simulink model "BestRun_VehicleModel_pntwo"  (R2021b)
settings: Solver=ode4  StartTime=0.0  StopTime=800  FixedStep=0.01  RelTol=1e-3  EnableMultiTasking=on
values from neighbouring files (symbols this model uses):
  Aera = 2.22    [Para_bestRun.m]
  BETT = 0.5*(0.878+0.844)*Mass*RofW    (= 426.1215567)    [Para_bestRun.m]
  Cd = 0.7153/Aera*0.8    (= 0.257765765766)    [Para_bestRun.m]
  deltM = 1+Yita+Iei*etaT/(Mass*RofW^2)*(gR0*[gRg1,gRg2,gRg3,gRg4,gRg5]).^2    [Para_bestRun.m]
  etaT = 0.92    [Para_bestRun.m]
  eTorq = self_MAPfilter(eTorq, 0.5)    [Load_BestRun_Parameters2.m]    (also in Para_bestRun.m = 1.1*[)
  fRoll = 0.1712/9.81    (= 0.0174515800204)    [Para_bestRun.m]
  gR0 = 3.863    [Para_bestRun.m]
  gRg1 = 3.620    (= 3.62)    [Para_bestRun.m]
  gRg2 = 1.925    [Para_bestRun.m]
  gRg3 = 1.285    [Para_bestRun.m]
  gRg4 = 0.936    [Para_bestRun.m]
  gRg5 = 0.667    [Para_bestRun.m]
  Iei = 0.211+0.001    (= 0.212)    [Para_bestRun.m]
  invMass = Mass    (= 1645)    [Para_bestRun.m]
  invThrAng = self_MAPfilter(invThrAng,0.5)    [Load_BestRun_Parameters2.m]
  Mass = 1645    [Para_bestRun.m]
  minTe = eTorq(:,1)    [Load_BestRun_Parameters2.m]
  minWe = eEngSpd    [Load_BestRun_Parameters2.m]
  N = 50    [par_test.m]    (also in run_simulink.m = vars.opt_N)
  pho = 1.29    [Para_bestRun.m]
  RofW = 0.98*0.307    (= 0.30086)    [Para_bestRun.m]
  Thr12 = [0 7.64 87.5 100]+Troffset    [Para_bestRun.m]
  Thr21 = [0 62.5 87.5 100]+Troffset    [Para_bestRun.m]
  Thr23 = [0 6.53 12.5 19.72 50 78.47 100]+Troffset    [Para_bestRun.m]
  Thr32 = [0 19.72 24.3 87.5 100]+Troffset    [Para_bestRun.m]
  Thr34 = [0 12.5 18.75 36.25 48.6 68 100]+Troffset    [Para_bestRun.m]
  Thr43 = [0 19.72 44.7 84.7 100]+Troffset    [Para_bestRun.m]
  Thr45 = [0 6.53 15.28 36.25 48.6 100]+Troffset    [Para_bestRun.m]
  Thr54 = [0 18.75 24.3 32.64 80.5 100]+Troffset    [Para_bestRun.m]
  Ts = 0.1    [par_test.m]    (also in run_simulink.m = vars.opt_Ts/100)
  V12 = [10 10 46.45 46.45]/3.6    [Para_bestRun.m]
  V21 = [8.3 8.3 38.3 38.3]/3.6    [Para_bestRun.m]
  V23 = [21.9 21.9 24.8 30.3 58.2 91.6 91.6]/3.6    [Para_bestRun.m]
  V32 = [8.3 8.3 20 83.3 83.3]/3.6    [Para_bestRun.m]
  V34 = [38.3 38.3 43.4 64.8 91.6 136.8 136.8]/3.6    [Para_bestRun.m]
  V43 = [24.8 24.8 60 110 110]/3.6    [Para_bestRun.m]
  V45 = [52.9 52.9  64.8 109.7 207.3 207.3]/3.6    [Para_bestRun.m]
  V54 = [49.7 49.7 52.9 64.8 189.4 189.4]/3.6    [Para_bestRun.m]
  wa = 0    [par_test.m]    (also in run_simulink.m = vars.opt_wa)
  wd = 1    [par_test.m]    (also in run_simulink.m = vars.opt_wd)
  wdu = 1    [par_test.m]    (also in run_simulink.m = vars.opt_wdu)
  wu = 4    [par_test.m]    (also in run_simulink.m = vars.opt_wu)
  wv = 0.01    [par_test.m]    (also in run_simulink.m = vars.opt_wv)
undefined symbols (not defined in the file or in its folder): N20, sfcFuelR
libraries: simulink x2
settings Model: Creator=Zhang Lei  LastModifiedBy=rlsot
settings SolverCC: AlgebraicLoopSolver=TrustRegion
settings DataIOCC: SaveFormat=Array  SignalLoggingSaveFormat=ModelDataLogs  SaveOutput=off  SaveTime=off  ReturnWorkspaceOutputs=off  SignalLoggingName=sigsOut
settings OptimizationCC: BlockReduction=off  OptimizeBlockIOStorage=off  BufferReuse=off  GlobalBufferReuse=off  ExpressionFolding=off  ExpressionDepthLimit=2147483647  LocalBlockOutputs=off  InitFltsAndDblsToZero=on  LifeSpan=inf  OptimizeDataStoreBuffers=off  BusAssignmentInplaceUpdate=off
settings DebuggingCC: AlgebraicLoopMsg=error  SaveWithParameterizedLinksMsg=none  UnderspecifiedInitializationDetection=Classic  MergeDetectMultiDrivingBlocksExec=none  SignalResolutionControl=TryResolveAllWithWarning  BlockPriorityViolationMsg=error  MinStepSizeMsg=error  MultiTaskDSMMsg=warning  MultiTaskCondExecSysMsg=none  MultiTaskRateTransMsg=warning  FcnCallInpInsideContextMsg=warning  StateNameClashWarn=warning  SFUnexpectedBacktrackingDiag=warning  SFNoUnconditionalDefaultTransitionDiag=warning  SFExecutionAtInitializationDiag=none  SFMachineParentedDataDiag=warning  ArithmeticOperatorsInVariantConditions=warning
settings HardwareCC: ProdBitPerPointer=32  ProdBitPerSizeT=32  ProdBitPerPtrDiffT=32  ProdLargestAtomicFloat=None  ProdWordSize=32  ProdLongLongMode=on  ProdHWDeviceType=Generic->32-bit x86 compatible
settings ModelReferenceCC: PropagateSignalLabelsOutOfModel=off
settings SFSimCC: SimUseLocalCustomCode=off  SimParseCustomCode=off  CustomCodeUndefinedFunction=UseInterfaceOnly
settings RTWCC: Description=Simulink Real-Time (OBSOLETE)  SystemTargetFile=slrt.tlc  TemplateMakefile=slrt_default_tmf  RTWUseLocalCustomCode=off  RTWCompilerOptimization=on
settings CodeAppCC: StateflowObjectComments=on
settings SimulinkRealTimeCC: TargetFcnLib=ansi_tfl_tmw.mat  CodeReplacementLibrary=None  MATLABClassNameForMDSCustomization=Simulink.SoftwareTarget.TargetSpecificTriggerConfigurationBase  xPCConcurrentTasks=on
settings ConfigComp: CovMetricSettings=dw  CovSaveCumulativeToWorkspaceVar=on  CovSaveSingleToWorkspaceVar=on  CovExternalEMLEnable=off  CovSFcnEnable=off

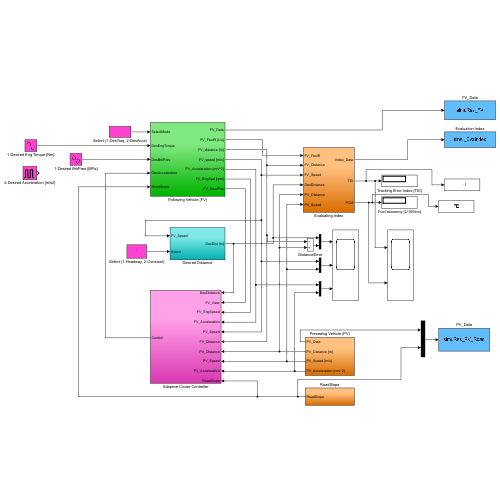
[thumbnail: Simulink's stored preview of the top-level diagram]
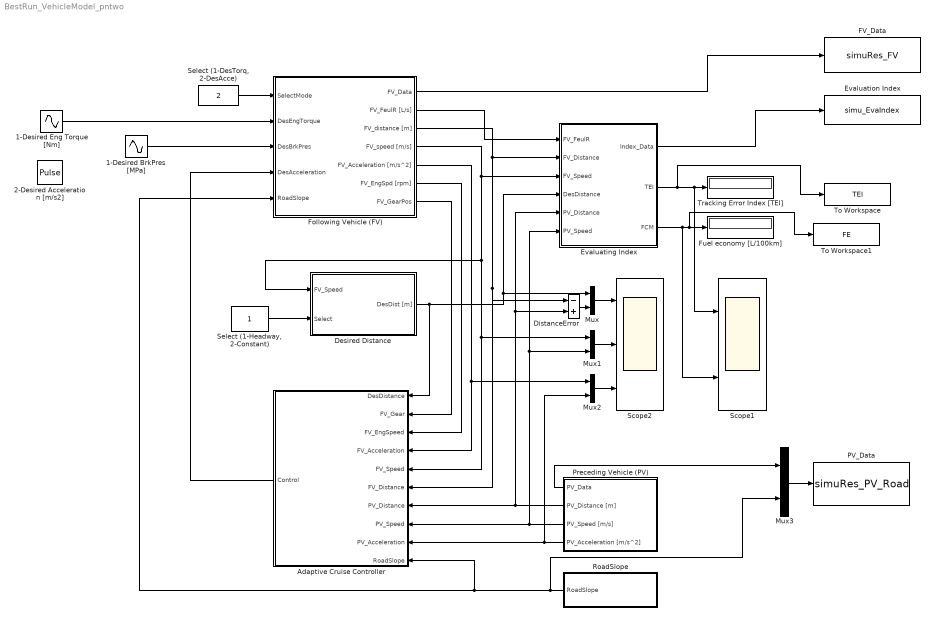
== system BestRun_VehicleModel_pntwo ==
  1-Desired BrkPres [MPa] : Sin  Amplitude=70  Bias=90  Frequency=2*pi*0.1  SampleTime=0
  1-Desired Eng Torque [Nm] : Sin  Amplitude=70  Bias=90  Frequency=2*pi*0.1  SampleTime=0
  2-Desired Acceleration [m/s2] : DiscretePulseGenerator  PulseType=Time based  Amplitude=0.6  Period=10  PulseWidth=50
  Adaptive Cruise Controller : Subsystem
  Desired Distance : Subsystem
  DistanceError : Sum  Inputs=-+
  Evaluating Index : Subsystem
  Evaluation Index : ToWorkspace  VariableName=simu_EvaIndex  SaveFormat=Structure With Time  SampleTime=-1
  FV_Data : ToWorkspace  VariableName=simuRes_FV  SaveFormat=Structure With Time  SampleTime=-1
  Following Vehicle (FV) : Subsystem
  Fuel economy [L/100km] : Display
  Mux{,1..3} (4 alike) : Mux  Inputs=2
  PV_Data : ToWorkspace  VariableName=simuRes_PV_Road  SaveFormat=Structure With Time  SampleTime=-1
  Preceding Vehicle (PV) : Subsystem
  RoadSlope : Subsystem
  Scope1 : Scope  NumInputPorts=2
  Scope2 : Scope  NumInputPorts=3
  "Select (1-DesTorq, 2-DesAcce)" : Constant  Value=2
  "Select (1-Headway, 2-Constant)" : Constant
  To Workspace : ToWorkspace  VariableName=TEI  SaveFormat=Timeseries  SampleTime=-1
  To Workspace1 : ToWorkspace  VariableName=FE  SaveFormat=Timeseries  SampleTime=-1
  Tracking Error Index [TEI] : Display
  wires:
  Following Vehicle (FV)/1(FV_Data) -> FV_Data/1
  1-Desired Eng Torque [Nm]/1 -> Following Vehicle (FV)/2(DesEngTorque)
  "Select (1-DesTorq, 2-DesAcce)"/1 -> Following Vehicle (FV)/1(SelectMode)
  Following Vehicle (FV)/7(FV_GearPos) -> Adaptive Cruise Controller/2(FV_Gear)
  Following Vehicle (FV)/6(FV_EngSpd [rpm]) -> Adaptive Cruise Controller/3(FV_EngSpeed)
  Following Vehicle (FV)/5(FV_Acceleration [m/s^2]) -> Adaptive Cruise Controller/4(FV_Acceleration), Mux2/1
  Following Vehicle (FV)/4(FV_speed [m/s]) -> Adaptive Cruise Controller/5(FV_Speed), Mux1/1, Desired Distance/1(FV_Speed), Evaluating Index/3(FV_Speed)
  Following Vehicle (FV)/3(FV_distance [m]) -> DistanceError/1, Adaptive Cruise Controller/6(FV_Distance), Evaluating Index/2(FV_Distance)
  Preceding Vehicle (PV)/2(PV_Distance [m]) -> DistanceError/2, Evaluating Index/5(PV_Distance), Adaptive Cruise Controller/7(PV_Distance)
  Preceding Vehicle (PV)/3(PV_Speed [m/s]) -> Adaptive Cruise Controller/8(PV_Speed), Evaluating Index/6(PV_Speed), Mux1/2
  Preceding Vehicle (PV)/4(PV_Acceleration [m/s^2]) -> Mux2/2, Adaptive Cruise Controller/9(PV_Acceleration)
  Mux/1 -> Scope2/1
  Mux1/1 -> Scope2/2
  Mux2/1 -> Scope2/3
  Adaptive Cruise Controller/1(Control) -> Following Vehicle (FV)/4(DesAcceleration)
  Desired Distance/1(DesDist [m]) -> Mux/1, Evaluating Index/4(DesDistance), Adaptive Cruise Controller/1(DesDistance)
  "Select (1-Headway, 2-Constant)"/1 -> Desired Distance/2(Select)
  Evaluating Index/3(FCM) -> To Workspace1/1, Fuel economy [L/100km]/1, Scope1/2
  Evaluating Index/2(TEI) -> To Workspace/1, Scope1/1, Tracking Error Index [TEI]/1
  Following Vehicle (FV)/2(FV_FeulR [L/s]) -> Evaluating Index/1(FV_FeulR)
  Evaluating Index/1(Index_Data) -> Evaluation Index/1
  1-Desired BrkPres [MPa]/1 -> Following Vehicle (FV)/3(DesBrkPres)
  RoadSlope/1(RoadSlope) -> Mux3/2, Following Vehicle (FV)/5(RoadSlope), Adaptive Cruise Controller/10(RoadSlope)
  Preceding Vehicle (PV)/1(PV_Data) -> Mux3/1
  Mux3/1 -> PV_Data/1
  DistanceError/1 -> Mux/2

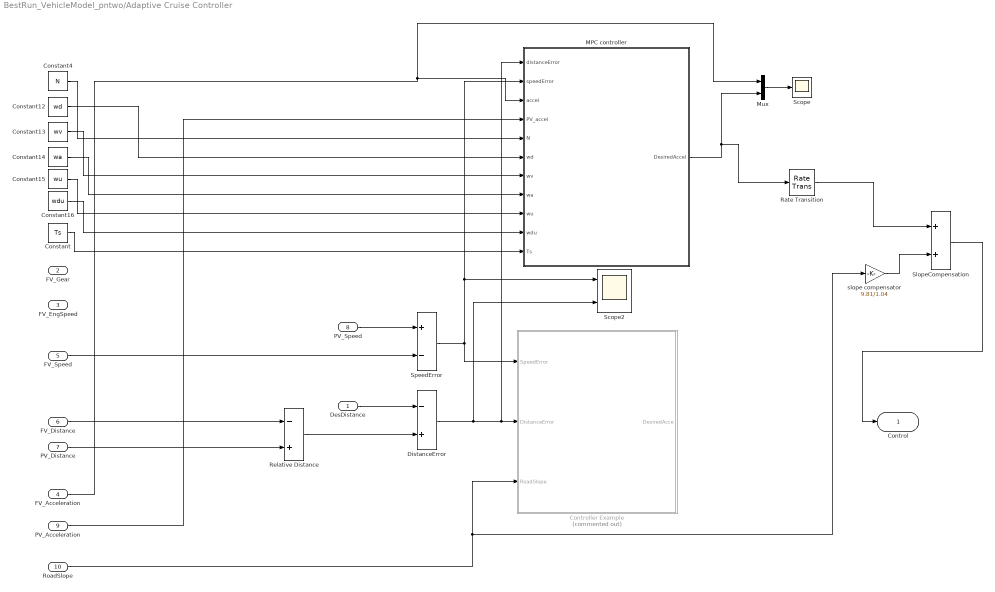
== system BestRun_VehicleModel_pntwo/Adaptive Cruise Controller ==
  DesDistance : Inport
  FV_Gear : Inport  Port=2
  FV_EngSpeed : Inport  Port=3
  FV_Acceleration : Inport  Port=4
  FV_Speed : Inport  Port=5
  FV_Distance : Inport  Port=6
  PV_Distance : Inport  Port=7
  PV_Speed : Inport  Port=8
  PV_Acceleration : Inport  Port=9
  RoadSlope : Inport  Port=10
  Constant : Constant  Value=Ts
  Constant12 : Constant  Value=wd  VectorParams1D=off
  Constant13 : Constant  Value=wv  VectorParams1D=off
  Constant14 : Constant  Value=wa  VectorParams1D=off
  Constant15 : Constant  Value=wu  VectorParams1D=off
  Constant16 : Constant  Value=wdu  VectorParams1D=off
  Constant4 : Constant  Value=N  VectorParams1D=off
  Controller Example : Subsystem  Commented=on
  DistanceError : Sum  Inputs=-+
  MPC controller : MATLAB Function  TreatAsAtomicUnit=on  SystemSampleTime=Ts
  Mux : Mux  Inputs=2
  Rate Transition : RateTransition  OutPortSampleTime=0.01
  Relative Distance : Sum  Inputs=-+
  Scope : Scope
  Scope2 : Scope  NumInputPorts=2
  SlopeCompensation : Sum
  SpeedError : Sum  Inputs=+-
  slope compensator : Gain  Gain=9.81/1.04
  Control : Outport  VectorParamsAs1DForOutWhenUnconnected=off
  wires:
  FV_Distance/1 -> Relative Distance/1
  PV_Distance/1 -> Relative Distance/2
  FV_Speed/1 -> SpeedError/2
  Relative Distance/1 -> DistanceError/2
  PV_Speed/1 -> SpeedError/1
  SpeedError/1 -> MPC controller/2(speedError), Scope2/1, Controller Example/1(SpeedError)
  DistanceError/1 -> Scope2/2, MPC controller/1(distanceError), Controller Example/2(DistanceError)
  DesDistance/1 -> DistanceError/1
  RoadSlope/1 -> slope compensator/1, Controller Example/3(RoadSlope)
  FV_Acceleration/1 -> Mux/1, MPC controller/3(accel)
  PV_Acceleration/1 -> MPC controller/4(PV_accel)
  MPC controller/1(DesiredAccel) -> Mux/2, Rate Transition/1
  Constant4/1 -> MPC controller/5(N)
  Mux/1 -> Scope/1
  Constant12/1 -> MPC controller/6(wd)
  Constant13/1 -> MPC controller/7(wv)
  Constant14/1 -> MPC controller/8(wa)
  Constant15/1 -> MPC controller/9(wu)
  Constant16/1 -> MPC controller/10(wdu)
  Constant/1 -> MPC controller/11(Ts)
  Rate Transition/1 -> SlopeCompensation/1
  slope compensator/1 -> SlopeCompensation/2
  SlopeCompensation/1 -> Control/1

== system BestRun_VehicleModel_pntwo/Desired Distance ==
  FV_Speed : Inport
  Select : Inport  Port=2
  Add : Sum
  Constant Distance : Constant  Value=45
  Headway Time : Gain  Gain=3
  MS : MultiPortSwitch  Inputs=2  SaturateOnIntegerOverflow=on
  Stop Distance : Constant  Value=15
  DesDist [m] : Outport  VectorParamsAs1DForOutWhenUnconnected=off
  wires:
  Stop Distance/1 -> Add/2
  FV_Speed/1 -> Headway Time/1
  Headway Time/1 -> Add/1
  Select/1 -> MS/1
  MS/1 -> DesDist [m]/1
  Add/1 -> MS/2
  Constant Distance/1 -> MS/3

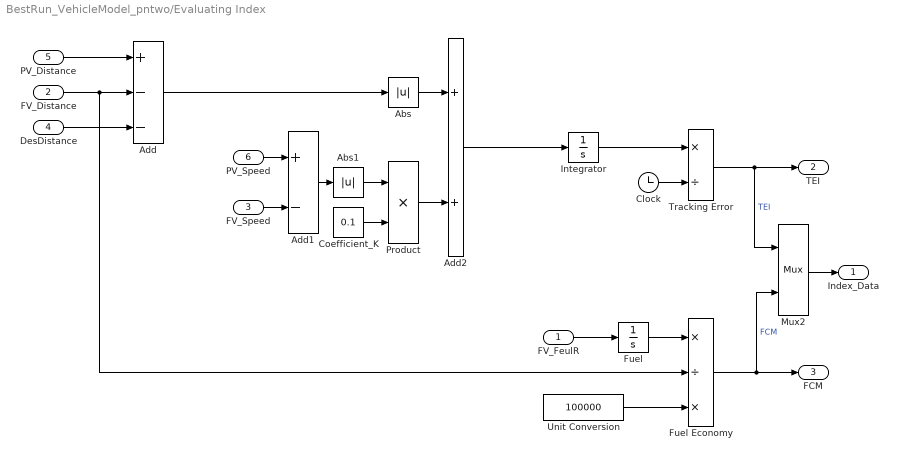
== system BestRun_VehicleModel_pntwo/Evaluating Index ==
  FV_FeulR : Inport
  FV_Distance : Inport  Port=2
  FV_Speed : Inport  Port=3
  DesDistance : Inport  Port=4
  PV_Distance : Inport  Port=5
  PV_Speed : Inport  Port=6
  Abs : Abs
  Abs1 : Abs
  Add : Sum  Inputs=+--
  Add1 : Sum  Inputs=+-
  Add2 : Sum
  Clock : Clock
  Coefficient_K : Constant  Value=0.1
  Fuel : Integrator
  Fuel Economy : Product  Inputs=*/*
  Integrator : Integrator
  Mux2 : Mux  Inputs=2
      settings: DisplayOption=signals
  Product : Product
  Tracking Error : Product  Inputs=*/
  Unit Conversion : Constant  Value=100000
  Index_Data : Outport  VectorParamsAs1DForOutWhenUnconnected=off
  TEI : Outport  Port=2  VectorParamsAs1DForOutWhenUnconnected=off
  FCM : Outport  Port=3  VectorParamsAs1DForOutWhenUnconnected=off
  wires:
  PV_Distance/1 -> Add/1
  FV_Distance/1 -> Fuel Economy/2, Add/2
  DesDistance/1 -> Add/3
  Add/1 -> Abs/1
  PV_Speed/1 -> Add1/1
  FV_Speed/1 -> Add1/2
  Add1/1 -> Abs1/1
  Abs1/1 -> Product/1
  Coefficient_K/1 -> Product/2
  Product/1 -> Add2/2
  Abs/1 -> Add2/1
  Add2/1 -> Integrator/1
  Integrator/1 -> Tracking Error/1
  Clock/1 -> Tracking Error/2
  FV_FeulR/1 -> Fuel/1
  Fuel/1 -> Fuel Economy/1
  Fuel Economy/1 -> Mux2/2, FCM/1  "FCM"
  Unit Conversion/1 -> Fuel Economy/3
  Mux2/1 -> Index_Data/1
  Tracking Error/1 -> Mux2/1, TEI/1  "TEI"

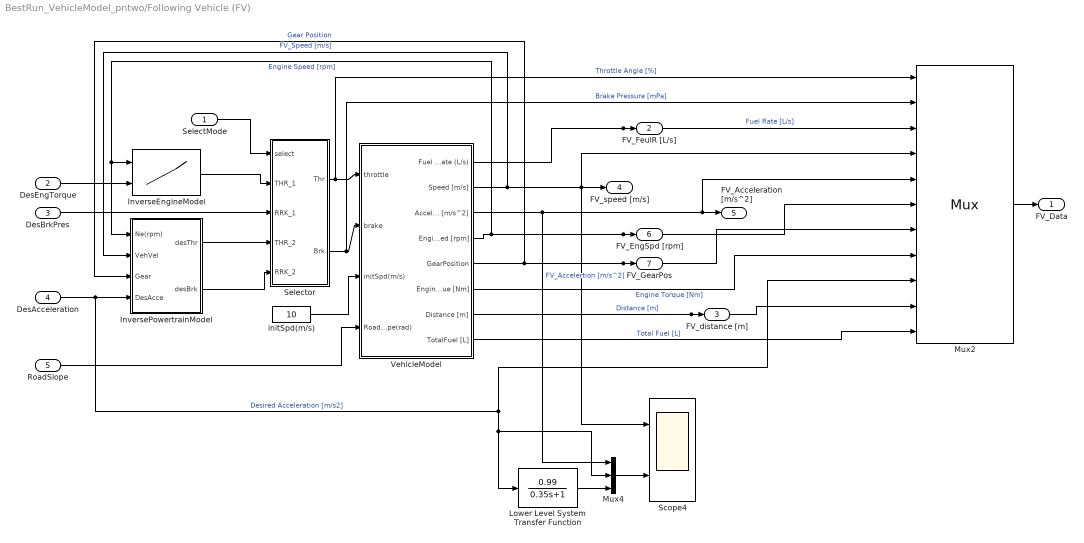
== system BestRun_VehicleModel_pntwo/Following Vehicle (FV) ==
  SelectMode : Inport
  DesEngTorque : Inport  Port=2
  DesBrkPres : Inport  Port=3
  DesAcceleration : Inport  Port=4
  RoadSlope : Inport  Port=5
  InverseEngineModel : Lookup2D  RowIndex=invWe  ColumnIndex=invTe  Table=invThrAng  LookUpMeth=Interpolation-Use End Values  SaturateOnIntegerOverflow=on
  InversePowertrainModel : Subsystem
  Lower Level System Transfer Function : TransferFcn  Numerator=[0.99]  Denominator=[0.35 1]
  Mux2 : Mux  Inputs=11
      settings: DisplayOption=signals
  Mux4 : Mux  Inputs=3
  Scope4 : Scope  NumInputPorts=2
  Selector : Subsystem
  VehicleModel : Subsystem
  initSpd(m/s) : Constant  Value=10
  FV_Data : Outport  VectorParamsAs1DForOutWhenUnconnected=off
  FV_FeulR [L/s] : Outport  Port=2  VectorParamsAs1DForOutWhenUnconnected=off
  FV_distance [m] : Outport  Port=3  VectorParamsAs1DForOutWhenUnconnected=off
  FV_speed [m/s] : Outport  Port=4  VectorParamsAs1DForOutWhenUnconnected=off
  FV_Acceleration [m/s^2] : Outport  Port=5  VectorParamsAs1DForOutWhenUnconnected=off
  FV_EngSpd [rpm] : Outport  Port=6  VectorParamsAs1DForOutWhenUnconnected=off
  FV_GearPos : Outport  Port=7  VectorParamsAs1DForOutWhenUnconnected=off
  wires:
  VehicleModel/6(EngineTorque [Nm]) -> Mux2/8  "Engine Torque [Nm]"
  VehicleModel/2(Speed [m/s]) -> InversePowertrainModel/2(VehVel), Mux2/4, FV_speed [m/s]/1, Scope4/1  "FV_Speed [m/s]"
  VehicleModel/1(Fuel Rate (L/s)) -> Mux2/3, FV_FeulR [L/s]/1  "Fuel Rate [L/s]"
  DesEngTorque/1 -> InverseEngineModel/2
  VehicleModel/4(EngineSpeed [rpm]) -> FV_EngSpd [rpm]/1, Mux2/6, InversePowertrainModel/1(Ne(rpm)), InverseEngineModel/1  "Engine Speed [rpm]"
  InverseEngineModel/1 -> Selector/2(THR_1)
  InversePowertrainModel/1(desThr) -> Selector/4(THR_2)
  DesAcceleration/1 -> InversePowertrainModel/4(DesAcce), Lower Level System Transfer Function/1, Mux4/2, Mux2/9  "Desired Acceleration [m/s2]"
  VehicleModel/5(GearPosition) -> Mux2/7, FV_GearPos/1, InversePowertrainModel/3(Gear)  "Gear Position"
  Selector/2(Brk) -> Mux2/2, VehicleModel/2(brake)  "Brake Pressure [mPa]"
  InversePowertrainModel/2(desBrk) -> Selector/5(RRK_2)
  Selector/1(Thr) -> Mux2/1, VehicleModel/1("throttle ")  "Throttle Angle [%]"
  VehicleModel/3(Acceleration [m/s^2]) -> Mux4/1, FV_Acceleration [m/s^2]/1, Mux2/5  "FV_Accelertion [m/s^2]"
  initSpd(m/s)/1 -> VehicleModel/3(initSpd(m/s))
  Lower Level System Transfer Function/1 -> Mux4/3
  Mux4/1 -> Scope4/2
  VehicleModel/7(Distance [m]) -> Mux2/10, FV_distance [m]/1  "Distance [m]"
  Mux2/1 -> FV_Data/1
  SelectMode/1 -> Selector/1(select)
  VehicleModel/8(TotalFuel [L]) -> Mux2/11  "Total Fuel [L]"
  DesBrkPres/1 -> Selector/3(RRK_1)
  RoadSlope/1 -> VehicleModel/4(RoadSlope(rad))

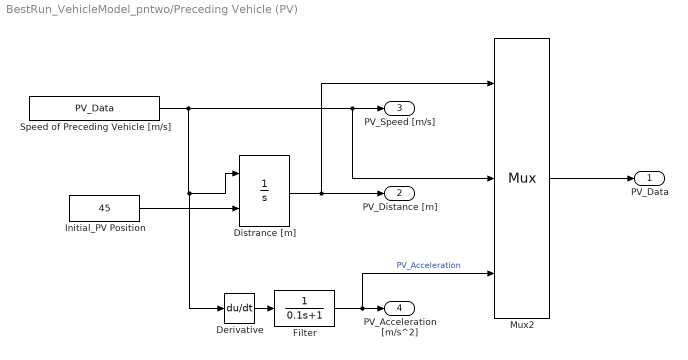
== system BestRun_VehicleModel_pntwo/Preceding Vehicle (PV) ==
  Derivative : Derivative
  Distrance [m] : Integrator  InitialConditionSource=external  InitialCondition=40  UpperSaturationLimit=100  LowerSaturationLimit=0.1
  Filter : TransferFcn  Denominator=[0.1 1]
  Initial_PV Position : Constant  Value=45
  Mux2 : Mux  Inputs=3
      settings: DisplayOption=signals
  Speed of Preceding Vehicle [m/s] : FromWorkspace  VariableName=PV_Data
  PV_Data : Outport  VectorParamsAs1DForOutWhenUnconnected=off
  PV_Distance [m] : Outport  Port=2  VectorParamsAs1DForOutWhenUnconnected=off
  PV_Speed [m/s] : Outport  Port=3  VectorParamsAs1DForOutWhenUnconnected=off
  PV_Acceleration [m/s^2] : Outport  Port=4  VectorParamsAs1DForOutWhenUnconnected=off
  wires:
  Distrance [m]/1 -> Mux2/1, PV_Distance [m]/1
  Derivative/1 -> Filter/1
  Speed of Preceding Vehicle [m/s]/1 -> Mux2/2, PV_Speed [m/s]/1, Derivative/1, Distrance [m]/1
  Filter/1 -> Mux2/3, PV_Acceleration [m/s^2]/1  "PV_Acceleration"
  Mux2/1 -> PV_Data/1
  Initial_PV Position/1 -> Distrance [m]/2

== system BestRun_VehicleModel_pntwo/RoadSlope ==
  Deg-->Rad : Gain  Gain=3.14/180
  RoadSlope [deg] : FromWorkspace  VariableName=Road_Data
  RoadSlope : Outport  VectorParamsAs1DForOutWhenUnconnected=off
  wires:
  Deg-->Rad/1 -> RoadSlope/1
  RoadSlope [deg]/1 -> Deg-->Rad/1

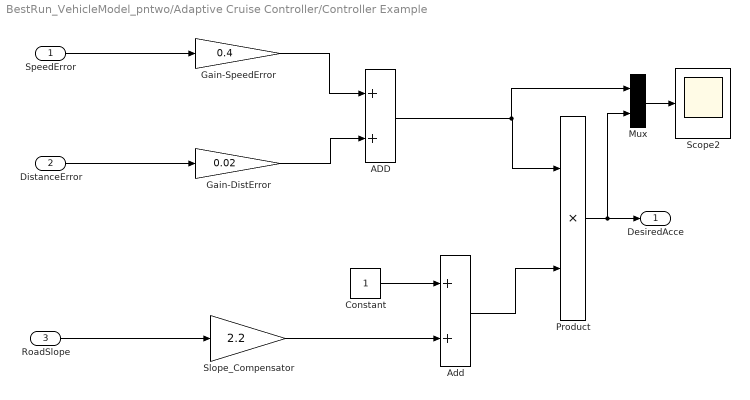
== system BestRun_VehicleModel_pntwo/Adaptive Cruise Controller/Controller Example ==
  SpeedError : Inport
  DistanceError : Inport  Port=2
  RoadSlope : Inport  Port=3
  ADD : Sum
  Add : Sum
  Constant : Constant
  Gain-DistError : Gain  Gain=0.02
  Gain-SpeedError : Gain  Gain=0.4
  Mux : Mux  Inputs=2
  Product : Product
  Scope2 : Scope
  Slope_Compensator : Gain  Gain=2.2
  DesiredAcce : Outport  VectorParamsAs1DForOutWhenUnconnected=off
  wires:
  Gain-DistError/1 -> ADD/2
  DistanceError/1 -> Gain-DistError/1
  SpeedError/1 -> Gain-SpeedError/1
  Gain-SpeedError/1 -> ADD/1
  Slope_Compensator/1 -> Add/2
  Product/1 -> Mux/2, DesiredAcce/1
  Add/1 -> Product/2
  RoadSlope/1 -> Slope_Compensator/1
  Constant/1 -> Add/1
  ADD/1 -> Mux/1, Product/1
  Mux/1 -> Scope2/1

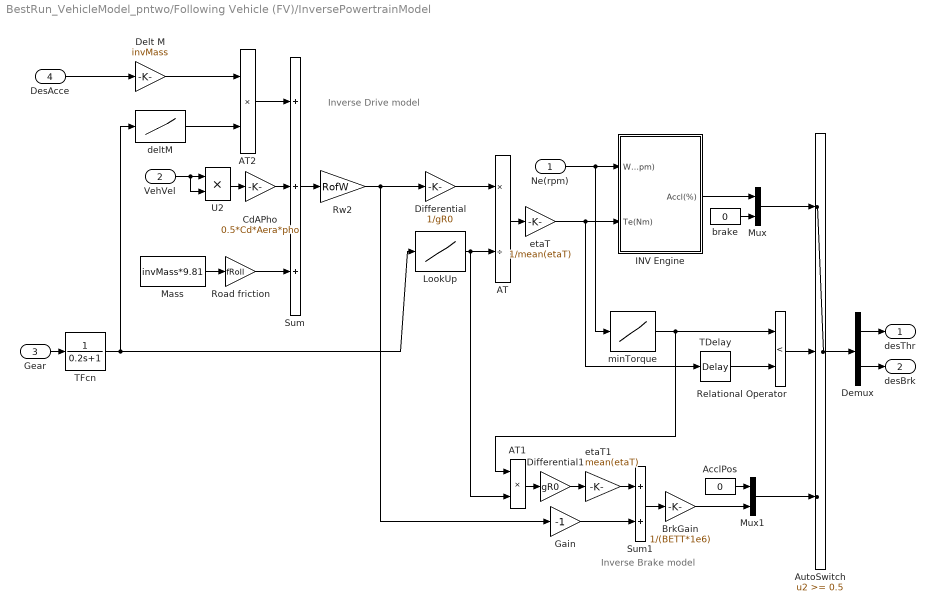
== system BestRun_VehicleModel_pntwo/Following Vehicle (FV)/InversePowertrainModel ==
  note: Inverse Drive model
  note: Inverse Brake model
  Ne(rpm) : Inport
  VehVel : Inport  Port=2
  Gear : Inport  Port=3
  DesAcce : Inport  Port=4
  AT : Product  Inputs=*/  InputSameDT=on  SaturateOnIntegerOverflow=on  OutDataTypeStr=Inherit: Same as first input
  AT1 : Product  Inputs=**  InputSameDT=on  SaturateOnIntegerOverflow=on  OutDataTypeStr=Inherit: Same as first input
  AT2 : Product  Inputs=**  InputSameDT=on  SaturateOnIntegerOverflow=on  OutDataTypeStr=Inherit: Same as first input
  AcclPos : Constant  Value=0
  AutoSwitch : Switch  Threshold=0.5
  BrkGain : Gain  Gain=1/(BETT*1e6)
  CdAPho : Gain  Gain=0.5*Cd*Aera*pho  SaturateOnIntegerOverflow=on  OutDataTypeStr=Inherit: Same as input  ParamDataTypeStr=Inherit: Same as input
  Delt M : Gain  Gain=invMass  SaturateOnIntegerOverflow=on  OutDataTypeStr=Inherit: Same as input  ParamDataTypeStr=Inherit: Same as input
  Demux : Demux  Outputs=2
  Differential : Gain  Gain=1/gR0  SaturateOnIntegerOverflow=on  OutDataTypeStr=Inherit: Same as input  ParamDataTypeStr=Inherit: Same as input
  Differential1 : Gain  Gain=gR0  SaturateOnIntegerOverflow=on  OutDataTypeStr=Inherit: Same as input  ParamDataTypeStr=Inherit: Same as input
  Gain : Gain  Gain=-1
  INV Engine : Subsystem
  LookUp : Lookup  InputValues=[0 1 2 3 4 5 6]  Table=[gRg1 gRg1 gRg2 gRg3 gRg4 gRg5 gRg5]  SaturateOnIntegerOverflow=on
  Mass : Constant  Value=invMass*9.81
  Mux : Mux  Inputs=2
  Mux1 : Mux  Inputs=2
  Relational Operator : RelationalOperator  Operator=<  OutDataTypeStr=boolean  RndMeth=Nearest
  Road friction : Gain  Gain=fRoll  SaturateOnIntegerOverflow=on  OutDataTypeStr=Inherit: Same as input  ParamDataTypeStr=Inherit: Same as input
  Rw2 : Gain  Gain=RofW  SaturateOnIntegerOverflow=on  OutDataTypeStr=Inherit: Same as input  ParamDataTypeStr=Inherit: Same as input
  Sum : Sum  Inputs=+++  SaturateOnIntegerOverflow=on
  Sum1 : Sum  Inputs=2  SaturateOnIntegerOverflow=on
  TDelay : TransportDelay  DelayTime=0.2
  TFcn : TransferFcn  Denominator=[0.2 1]
  U2 : Product  InputSameDT=on  SaturateOnIntegerOverflow=on  OutDataTypeStr=Inherit: Same as first input
  brake : Constant  Value=0
  deltM : Lookup  InputValues=[1 2 3 4 5]  Table=deltM  SaturateOnIntegerOverflow=on
  etaT : Gain  Gain=1/mean(etaT)  SaturateOnIntegerOverflow=on  OutDataTypeStr=Inherit: Same as input  ParamDataTypeStr=Inherit: Same as input
  etaT1 : Gain  Gain=mean(etaT)  SaturateOnIntegerOverflow=on  OutDataTypeStr=Inherit: Same as input  ParamDataTypeStr=Inherit: Same as input
  minTorque : Lookup  InputValues=minWe  Table=minTe  LookUpMeth=Interpolation-Use End Values  SaturateOnIntegerOverflow=on
  desThr : Outport  VectorParamsAs1DForOutWhenUnconnected=off
  desBrk : Outport  Port=2  VectorParamsAs1DForOutWhenUnconnected=off
  wires:
  CdAPho/1 -> Sum/2
  Road friction/1 -> Sum/3
  Mass/1 -> Road friction/1
  U2/1 -> CdAPho/1
  VehVel/1 -> U2/1, U2/2
  DesAcce/1 -> Delt M/1
  Gear/1 -> TFcn/1
  AT/1 -> etaT/1
  Sum/1 -> Rw2/1
  Rw2/1 -> Differential/1, Gain/1
  LookUp/1 -> AT/2, AT1/2
  etaT/1 -> INV Engine/2(Te(Nm)), TDelay/1
  Ne(rpm)/1 -> INV Engine/1(We(rpm)), minTorque/1
  Mux/1 -> AutoSwitch/1
  INV Engine/1(Accl(%)) -> Mux/1
  brake/1 -> Mux/2
  AutoSwitch/1 -> Demux/1
  Demux/1 -> desThr/1
  Demux/2 -> desBrk/1
  AcclPos/1 -> Mux1/1
  Mux1/1 -> AutoSwitch/3
  Sum1/1 -> BrkGain/1
  minTorque/1 -> Relational Operator/1, AT1/1
  Gain/1 -> Sum1/2
  Relational Operator/1 -> AutoSwitch/2
  Differential1/1 -> etaT1/1
  etaT1/1 -> Sum1/1
  AT1/1 -> Differential1/1
  TDelay/1 -> Relational Operator/2
  BrkGain/1 -> Mux1/2
  Differential/1 -> AT/1
  AT2/1 -> Sum/1
  Delt M/1 -> AT2/1
  deltM/1 -> AT2/2
  TFcn/1 -> LookUp/1, deltM/1

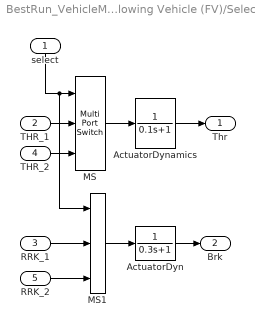
== system BestRun_VehicleModel_pntwo/Following Vehicle (FV)/Selector ==
  select : Inport
  THR_1 : Inport  Port=2
  RRK_1 : Inport  Port=3
  THR_2 : Inport  Port=4
  RRK_2 : Inport  Port=5
  ActuatorDyn : TransferFcn  Numerator=1  Denominator=[0.3 1]
  ActuatorDynamics : TransferFcn  Denominator=[0.1 1]
  MS : MultiPortSwitch  Inputs=2  SaturateOnIntegerOverflow=on
  MS1 : MultiPortSwitch  Inputs=2  SaturateOnIntegerOverflow=on
  Thr : Outport  VectorParamsAs1DForOutWhenUnconnected=off
  Brk : Outport  Port=2  VectorParamsAs1DForOutWhenUnconnected=off
  wires:
  RRK_2/1 -> MS1/3
  MS/1 -> ActuatorDynamics/1
  MS1/1 -> ActuatorDyn/1
  ActuatorDynamics/1 -> Thr/1
  ActuatorDyn/1 -> Brk/1
  select/1 -> MS1/1, MS/1
  THR_1/1 -> MS/2
  RRK_1/1 -> MS1/2
  THR_2/1 -> MS/3

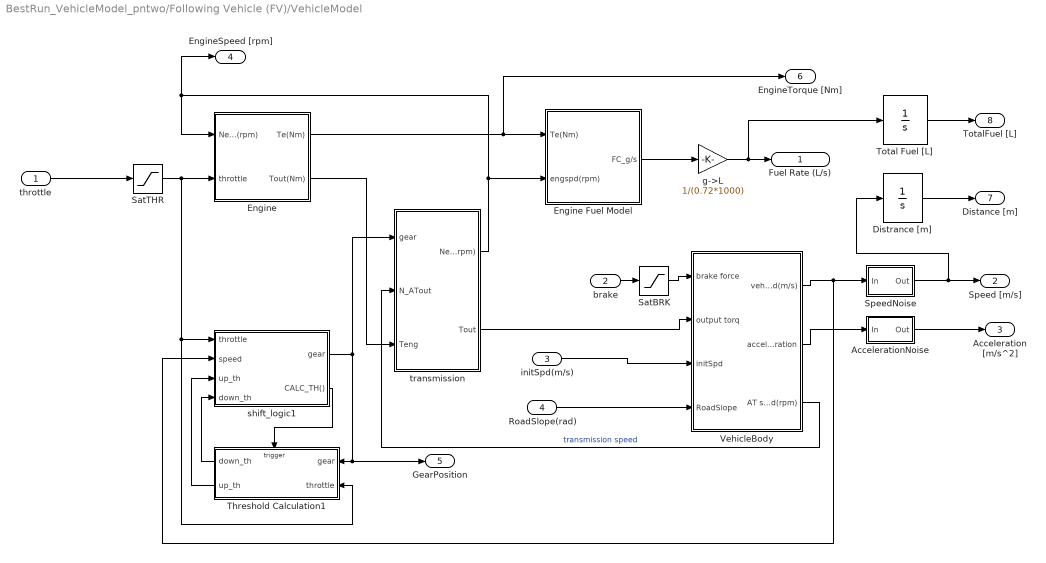
== system BestRun_VehicleModel_pntwo/Following Vehicle (FV)/VehicleModel ==
  "throttle " : Inport
  brake : Inport  Port=2
  initSpd(m/s) : Inport  Port=3
  RoadSlope(rad) : Inport  Port=4
  AccelerationNoise : Subsystem
  Distrance [m] : Integrator  UpperSaturationLimit=100  LowerSaturationLimit=0.1
  Engine : Subsystem
  Engine Fuel Model : Subsystem
  SatBRK : Saturate  UpperLimit=8  LowerLimit=0
  SatTHR : Saturate  UpperLimit=100  LowerLimit=0
  SpeedNoise : Subsystem
  Threshold Calculation1 : Subsystem  TreatAsAtomicUnit=on
  Total Fuel [L] : Integrator  UpperSaturationLimit=100  LowerSaturationLimit=0.1
  VehicleBody : Subsystem
  g->L : Gain  Gain=1/(0.72*1000)
  shift_logic1 : Stateflow chart  TreatAsAtomicUnit=on
  transmission : Subsystem
  Fuel Rate (L/s) : Outport  VectorParamsAs1DForOutWhenUnconnected=off
  Speed [m/s] : Outport  Port=2  VectorParamsAs1DForOutWhenUnconnected=off
  Acceleration [m/s^2] : Outport  Port=3  VectorParamsAs1DForOutWhenUnconnected=off
  EngineSpeed [rpm] : Outport  Port=4  VectorParamsAs1DForOutWhenUnconnected=off
  GearPosition : Outport  Port=5  VectorParamsAs1DForOutWhenUnconnected=off
  EngineTorque [Nm] : Outport  Port=6  VectorParamsAs1DForOutWhenUnconnected=off
  Distance [m] : Outport  Port=7  VectorParamsAs1DForOutWhenUnconnected=off
  TotalFuel [L] : Outport  Port=8  VectorParamsAs1DForOutWhenUnconnected=off
  wires:
  VehicleBody/3(AT speed(rpm)) -> transmission/2(N_ATout)  "transmission speed"
  Threshold Calculation1/1(down_th) -> shift_logic1/4(down_th)
  Threshold Calculation1/2(up_th) -> shift_logic1/3(up_th)
  shift_logic1/2(CALC_TH()) -> Threshold Calculation1/Trigger
  VehicleBody/1(vehSpd(m/s)) -> SpeedNoise/1(In), shift_logic1/2(speed)
  transmission/2(Tout) -> VehicleBody/2(output torq)
  transmission/1(Neng(rpm)) -> Engine/1(Neng(rpm)), EngineSpeed [rpm]/1, Engine Fuel Model/2(engspd(rpm))
  brake/1 -> SatBRK/1
  "throttle "/1 -> SatTHR/1
  shift_logic1/1(gear) -> transmission/1(gear), Threshold Calculation1/1(gear), GearPosition/1
  SatTHR/1 -> Engine/2(throttle), shift_logic1/1(throttle), Threshold Calculation1/2(throttle)
  SatBRK/1 -> VehicleBody/1(brake force)
  VehicleBody/2(acceleration) -> AccelerationNoise/1(In)
  Engine/1(Te(Nm)) -> EngineTorque [Nm]/1, Engine Fuel Model/1("Te(Nm) ")
  initSpd(m/s)/1 -> VehicleBody/3(initSpd)
  Engine/2(Tout(Nm)) -> transmission/3(Teng)
  SpeedNoise/1(Out) -> Distrance [m]/1, Speed [m/s]/1
  AccelerationNoise/1(Out) -> Acceleration [m/s^2]/1
  Engine Fuel Model/1(FC_g/s) -> g->L/1
  g->L/1 -> Total Fuel [L]/1, Fuel Rate (L/s)/1
  Distrance [m]/1 -> Distance [m]/1
  Total Fuel [L]/1 -> TotalFuel [L]/1
  RoadSlope(rad)/1 -> VehicleBody/4(RoadSlope)

== system BestRun_VehicleModel_pntwo/Following Vehicle (FV)/InversePowertrainModel/INV Engine ==
  We(rpm) : Inport
  Te(Nm) : Inport  Port=2
  InverseTe : Lookup2D  RowIndex=invWe  ColumnIndex=invTe  Table=invThrAng  LookUpMeth=Interpolation-Use End Values  SaturateOnIntegerOverflow=on
  Accl(%) : Outport  VectorParamsAs1DForOutWhenUnconnected=off
  wires:
  We(rpm)/1 -> InverseTe/1
  Te(Nm)/1 -> InverseTe/2
  InverseTe/1 -> Accl(%)/1

== system BestRun_VehicleModel_pntwo/Following Vehicle (FV)/VehicleModel/AccelerationNoise ==
  In : Inport
  Sum : Sum  Inputs=|++  SaturateOnIntegerOverflow=on
  Transfer Fcn : TransferFcn  Denominator=[0.05 1]
  White Noise : simulink/Sources/Band-Limited White Noise  Cov=[0.000005]  Ts=0.01  seed=[231]
  Out : Outport  VectorParamsAs1DForOutWhenUnconnected=off
  wires:
  In/1 -> Sum/2
  Sum/1 -> Out/1
  White Noise/1 -> Transfer Fcn/1
  Transfer Fcn/1 -> Sum/1

== system BestRun_VehicleModel_pntwo/Following Vehicle (FV)/VehicleModel/Engine ==
  Neng(rpm) : Inport
  throttle : Inport  Port=2
  Diff : Derivative
  Sum : Sum  Inputs=-+  InputSameDT=on  SaturateOnIntegerOverflow=on  OutDataTypeStr=Inherit: Same as first input
  Transfer Fcn : TransferFcn  Denominator=[0.3 1]
  engine torque : Lookup2D  RowIndex=eEngSpd  ColumnIndex=eThrAng  Table=eTorq  LookUpMeth=Interpolation-Use End Values  SaturateOnIntegerOverflow=on  InputSameDT=on
  engine + impeller inertia2 : Gain  Gain=Iei  SaturateOnIntegerOverflow=on  OutDataTypeStr=Inherit: Same as input  ParamDataTypeStr=Inherit: Same as input
  to RPM : Gain  Gain=pi/30  SaturateOnIntegerOverflow=on  OutDataTypeStr=Inherit: Same as input  ParamDataTypeStr=Inherit: Same as input
  Te(Nm) : Outport  InitialOutput=0  VectorParamsAs1DForOutWhenUnconnected=off
  Tout(Nm) : Outport  Port=2  InitialOutput=0  VectorParamsAs1DForOutWhenUnconnected=off
  wires:
  Neng(rpm)/1 -> engine torque/1, to RPM/1
  engine torque/1 -> Transfer Fcn/1
  Transfer Fcn/1 -> Sum/2, Te(Nm)/1
  throttle/1 -> engine torque/2
  engine + impeller inertia2/1 -> Sum/1
  Diff/1 -> engine + impeller inertia2/1
  to RPM/1 -> Diff/1
  Sum/1 -> Tout(Nm)/1

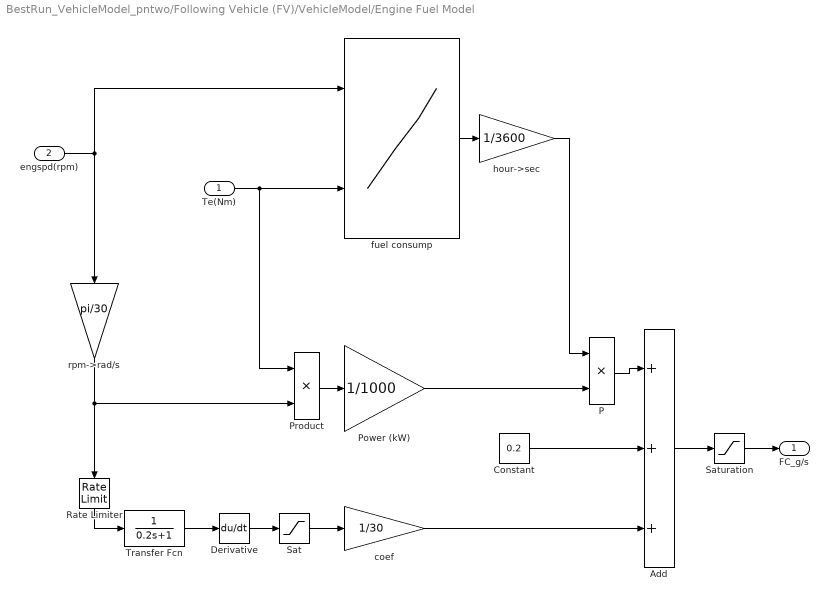
== system BestRun_VehicleModel_pntwo/Following Vehicle (FV)/VehicleModel/Engine Fuel Model ==
  "Te(Nm) " : Inport
  engspd(rpm) : Inport  Port=2
  Add : Sum  Inputs=+++
  Constant : Constant  Value=0.2
  Derivative : Derivative
  P : Product  RndMeth=Zero
  Power (kW) : Gain  Gain=1/1000
  Product : Product  RndMeth=Zero
  Rate Limiter : RateLimiter  RisingSlewLimit=50  FallingSlewLimit=-50  SampleTimeMode=inherited
  Sat : Saturate  UpperLimit=5  LowerLimit=0
  Saturation : Saturate  UpperLimit=inf  LowerLimit=0
  Transfer Fcn : TransferFcn  Denominator=[0.2 1]
  coef : Gain  Gain=1/30
  fuel consump : Lookup2D  RowIndex=sfcWe  ColumnIndex=sfcTe  Table=sfcFuelR  LookUpMeth=Interpolation-Use End Values  SaturateOnIntegerOverflow=on  InputSameDT=on
  hour->sec : Gain  Gain=1/3600
  rpm->rad/s : Gain  Gain=pi/30
  FC_g/s : Outport  VectorParamsAs1DForOutWhenUnconnected=off
  wires:
  engspd(rpm)/1 -> fuel consump/1, rpm->rad/s/1
  "Te(Nm) "/1 -> fuel consump/2, Product/1
  fuel consump/1 -> hour->sec/1
  Product/1 -> Power (kW)/1
  Power (kW)/1 -> P/2
  hour->sec/1 -> P/1
  rpm->rad/s/1 -> Rate Limiter/1, Product/2
  Saturation/1 -> FC_g/s/1
  P/1 -> Add/1
  Add/1 -> Saturation/1
  Constant/1 -> Add/2
  Derivative/1 -> Sat/1
  Transfer Fcn/1 -> Derivative/1
  Rate Limiter/1 -> Transfer Fcn/1
  coef/1 -> Add/3
  Sat/1 -> coef/1

== system BestRun_VehicleModel_pntwo/Following Vehicle (FV)/VehicleModel/SpeedNoise ==
  In : Inport
  Sum : Sum  Inputs=|++  SaturateOnIntegerOverflow=on
  Transfer Fcn : TransferFcn  Denominator=[0.05 1]
  White Noise : simulink/Sources/Band-Limited White Noise  Cov=[0.0003]  Ts=0.01  seed=[23341]
  Out : Outport  VectorParamsAs1DForOutWhenUnconnected=off
  wires:
  White Noise/1 -> Transfer Fcn/1
  Sum/1 -> Out/1
  In/1 -> Sum/2
  Transfer Fcn/1 -> Sum/1

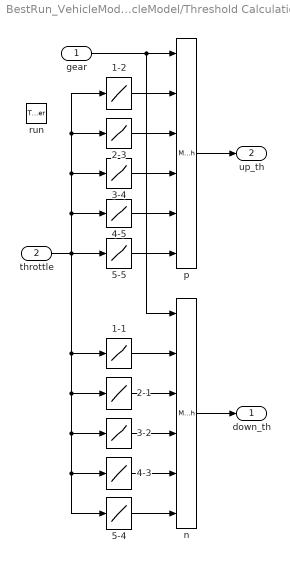
== system BestRun_VehicleModel_pntwo/Following Vehicle (FV)/VehicleModel/Threshold Calculation1 ==
  gear : Inport
  throttle : Inport  Port=2
  run : TriggerPort  TriggerType=function-call  VariantControl=(inherit)
  1-1 : Lookup  InputValues=[0 100]  Table=[0 0]  SaturateOnIntegerOverflow=on
  1-2 : Lookup  InputValues=Thr12  Table=V12  SaturateOnIntegerOverflow=on
  2-1 : Lookup  InputValues=Thr21  Table=V21  SaturateOnIntegerOverflow=on
  2-3 : Lookup  InputValues=Thr23  Table=V23  SaturateOnIntegerOverflow=on
  3-2 : Lookup  InputValues=Thr32  Table=V32  SaturateOnIntegerOverflow=on
  3-4 : Lookup  InputValues=Thr34  Table=V34  SaturateOnIntegerOverflow=on
  4-3 : Lookup  InputValues=Thr43  Table=V43  SaturateOnIntegerOverflow=on
  4-5 : Lookup  InputValues=Thr45  Table=V45  SaturateOnIntegerOverflow=on
  5-4 : Lookup  InputValues=Thr54  Table=V54  SaturateOnIntegerOverflow=on
  5-5 : Lookup  InputValues=[0 100]  Table=[1000 1000]  SaturateOnIntegerOverflow=on
  n : MultiPortSwitch  Inputs=5  SaturateOnIntegerOverflow=on  InputSameDT=on
  p : MultiPortSwitch  Inputs=5  SaturateOnIntegerOverflow=on  InputSameDT=on
  down_th : Outport  VectorParamsAs1DForOutWhenUnconnected=off
  up_th : Outport  Port=2  VectorParamsAs1DForOutWhenUnconnected=off
  wires:
  n/1 -> down_th/1
  p/1 -> up_th/1
  throttle/1 -> 4-5/1, 3-4/1, 2-3/1, 1-2/1, 3-2/1, 4-3/1, 5-4/1, 2-1/1, 1-1/1, 5-5/1
  4-3/1 -> n/5
  3-2/1 -> n/4
  2-1/1 -> n/3
  1-1/1 -> n/2
  gear/1 -> n/1, p/1
  4-5/1 -> p/5
  3-4/1 -> p/4
  2-3/1 -> p/3
  1-2/1 -> p/2
  5-5/1 -> p/6
  5-4/1 -> n/6

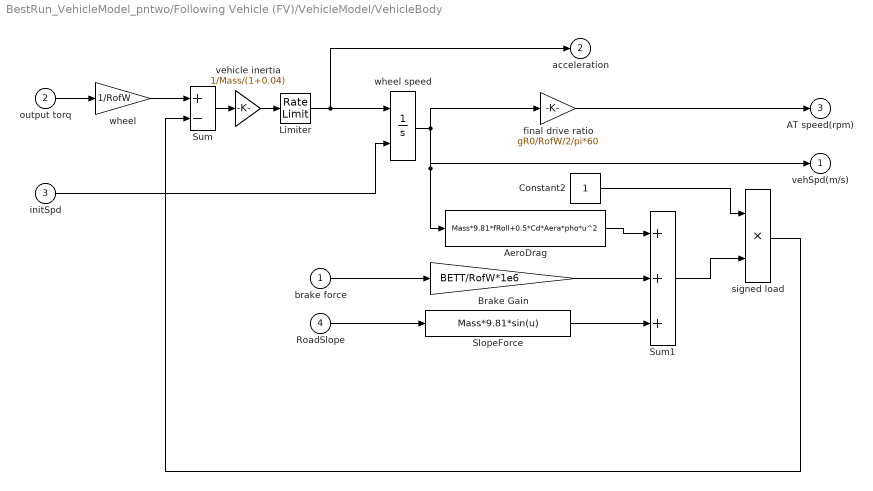
== system BestRun_VehicleModel_pntwo/Following Vehicle (FV)/VehicleModel/VehicleBody ==
  brake force : Inport
  output torq : Inport  Port=2
  initSpd : Inport  Port=3
  RoadSlope : Inport  Port=4
  AeroDrag : Fcn  Expr=Mass*9.81*fRoll+0.5*Cd*Aera*pho*u^2
  Brake Gain : Gain  Gain=BETT/RofW*1e6  SaturateOnIntegerOverflow=on  OutDataTypeStr=Inherit: Same as input  ParamDataTypeStr=Inherit: Same as input
  Constant2 : Constant
  Limiter : RateLimiter  RisingSlewLimit=1.5  FallingSlewLimit=-1.5
  SlopeForce : Fcn  Expr=Mass*9.81*sin(u)
  Sum : Sum  Inputs=+-  InputSameDT=on  SaturateOnIntegerOverflow=on  OutDataTypeStr=Inherit: Same as first input
  Sum1 : Sum  Inputs=+++  InputSameDT=on  SaturateOnIntegerOverflow=on  OutDataTypeStr=Inherit: Same as first input
  final drive ratio : Gain  Gain=gR0/RofW/2/pi*60  SaturateOnIntegerOverflow=on  OutDataTypeStr=Inherit: Same as input  ParamDataTypeStr=Inherit: Same as input
  signed load : Product  InputSameDT=on  SaturateOnIntegerOverflow=on  OutDataTypeStr=Inherit: Same as first input
  vehicle inertia : Gain  Gain=1/Mass/(1+0.04)  SaturateOnIntegerOverflow=on  OutDataTypeStr=Inherit: Same as input  ParamDataTypeStr=Inherit: Same as input
  wheel : Gain  Gain=1/RofW  SaturateOnIntegerOverflow=on  OutDataTypeStr=Inherit: Same as input  ParamDataTypeStr=Inherit: Same as input
  wheel speed : Integrator  InitialConditionSource=external  InitialCondition=N20  LimitOutput=on  UpperSaturationLimit=100  LowerSaturationLimit=0.1
  vehSpd(m/s) : Outport  InitialOutput=0  VectorParamsAs1DForOutWhenUnconnected=off
  acceleration : Outport  Port=2  InitialOutput=0  VectorParamsAs1DForOutWhenUnconnected=off
  AT speed(rpm) : Outport  Port=3  InitialOutput=0  VectorParamsAs1DForOutWhenUnconnected=off
  wires:
  final drive ratio/1 -> AT speed(rpm)/1
  brake force/1 -> Brake Gain/1
  Sum1/1 -> signed load/2
  AeroDrag/1 -> Sum1/1
  signed load/1 -> Sum/2
  output torq/1 -> wheel/1
  vehicle inertia/1 -> Limiter/1
  Sum/1 -> vehicle inertia/1
  wheel speed/1 -> final drive ratio/1, vehSpd(m/s)/1, AeroDrag/1
  Constant2/1 -> signed load/1
  initSpd/1 -> wheel speed/2
  wheel/1 -> Sum/1
  Brake Gain/1 -> Sum1/2
  Limiter/1 -> acceleration/1, wheel speed/1
  RoadSlope/1 -> SlopeForce/1
  SlopeForce/1 -> Sum1/3

== system BestRun_VehicleModel_pntwo/Following Vehicle (FV)/VehicleModel/transmission ==
  gear : Inport
  N_ATout : Inport  Port=2
  Teng : Inport  Port=3
  First Order sys : Subsystem  mask{T=0.2, initX=2000}
      mask prompts: T "Const Time"; initX "initial state"
  Sat_engSpd : Saturate  UpperLimit=6500  LowerLimit=800
  efficiency : Gain  Gain=etaT  SaturateOnIntegerOverflow=on  OutDataTypeStr=Inherit: Same as input  ParamDataTypeStr=Inherit: Same as input
  final gear : Gain  Gain=gR0  SaturateOnIntegerOverflow=on  OutDataTypeStr=Inherit: Same as input  ParamDataTypeStr=Inherit: Same as input
  transmission ratio : Subsystem
  Neng(rpm) : Outport  InitialOutput=0  VectorParamsAs1DForOutWhenUnconnected=off
  Tout : Outport  Port=2  InitialOutput=0  VectorParamsAs1DForOutWhenUnconnected=off
  wires:
  transmission ratio/1(Tout) -> efficiency/1
  N_ATout/1 -> transmission ratio/3(Nout)
  transmission ratio/2(Nin) -> Sat_engSpd/1
  gear/1 -> transmission ratio/2(gear)
  Teng/1 -> transmission ratio/1(Tin)  "turbine torque"
  efficiency/1 -> final gear/1
  final gear/1 -> Tout/1
  Sat_engSpd/1 -> First Order sys/1(u)
  First Order sys/1(x) -> Neng(rpm)/1

== system BestRun_VehicleModel_pntwo/Following Vehicle (FV)/VehicleModel/transmission/First Order sys ==
  u : Inport
  State-Space : StateSpace  A=-1/T  B=1/T  D=0  InitialCondition=initX
  x : Outport  VectorParamsAs1DForOutWhenUnconnected=off
  wires:
  State-Space/1 -> x/1
  u/1 -> State-Space/1

== system BestRun_VehicleModel_pntwo/Following Vehicle (FV)/VehicleModel/transmission/transmission ratio ==
  Tin : Inport
  gear : Inport  Port=2
  Nout : Inport  Port=3
  Look-Up Table : Lookup  InputValues=[1 2 3 4 5]  Table=[gRg1 gRg2 gRg3 gRg4 gRg5]  SaturateOnIntegerOverflow=on
  Product : Product  InputSameDT=on  SaturateOnIntegerOverflow=on  OutDataTypeStr=Inherit: Same as first input
  Product1 : Product  InputSameDT=on  SaturateOnIntegerOverflow=on  OutDataTypeStr=Inherit: Same as first input
  Tout : Outport  InitialOutput=0  VectorParamsAs1DForOutWhenUnconnected=off
  Nin : Outport  Port=2  InitialOutput=0  VectorParamsAs1DForOutWhenUnconnected=off
  wires:
  Look-Up Table/1 -> Product/2, Product1/1
  Nout/1 -> Product1/2
  Product1/1 -> Nin/1
  Product/1 -> Tout/1
  Tin/1 -> Product/1
  gear/1 -> Look-Up Table/1

== matlab function BestRun_VehicleModel_pntwo/Adaptive Cruise Controller/MPC controller ==
  data: distanceError input; speedError input; DesiredAccel output; accel input; PV_accel input; N input; wd input; wv input; wa input; wu input; wdu input; Ts input
function DesiredAccel = fcn(distanceError,speedError,accel,PV_accel,N, wd,wv,wa,wu,wdu, Ts)
    % load MPC parameters CYH
    tau_h = 3; %名义时距
    T_L = 0.35;  K_L = 0.99;  %一阶惯性系统时间常数
    Phi = [0,1,-tau_h;0,0,-1;0,0,-1/T_L];
    Pi = [0;0;K_L/T_L];
    Gamma = [0;1;0];
    %状态空间离散化
    coder.extrinsic('c2d')
    [A,B] = c2d(Phi,Pi,Ts);
    [~,G] = c2d(Phi,Gamma,Ts);
    
    %求系数矩阵
    S1 = zeros(3*N,N);
    S2 = zeros(3*N,N);
    T = zeros(3*N,3);
    S1(1:3,1) = B;
    S2(1:3,1) = G;
    T(1:3,1:3) = A;
    for i=2:N
        S1(3*i-2:3*i,:) = A*S1(3*i-5:3*i-3,:);
        S1(3*i-2:3*i,i) = B;
        S2(3*i-2:3*i,:) = A*S2(3*i-5:3*i-3,:);
        S2(3*i-2:3*i,i) = G;
        T(3*i-2:3*i,:) = A*T(3*i-5:3*i-3,:);
    end
    
    
    D = zeros(N-1,N); %差分矩阵
    for i=1:N-1
        D(i,i) = -1;
        D(i,i+1) = 1;
    end
    
    %约束
    lbu = -1.5*ones(N,1);  %控制量下界，待定
    ubu = 1*ones(N,1);   %控制量上界，待定
    xmax = [10;5;1];      %状态量上界，待定
    xmin = [-10;-5;-1.5];   %状态量下界，待定
    dumax = 1;           %控制量导数上界，待定
    dumin = -1.5;          %控制量导数下界，待定
    %约束处理
    X1 = zeros(3*N,1);
    X2 = zeros(3*N,1);
    dU1 = dumin*ones(N-1,1);
    dU2 = dumax*ones(N-1,1);
    for i=1:N
        X1(3*i-2:3*i,1) = xmin;
        X2(3*i-2:3*i,1) = xmax;
    end
    %初始量
    x0 = [distanceError;speedError;accel];
    ap = PV_accel;
    V = ap*ones(N,1);

    %标准化约束系数矩阵
    Aeq = [];
    beq = [];
    A1 = [S1;-S1;D;-D];
    b1 = [X2-T*x0-S2*V;-(X1-T*x0-S2*V);dU2;-dU1];
    
   
    Q = zeros(3*N,3*N);
    for i=1:N
        Q(3*i-2:3*i,3*i-2:3*i) = diag([wd,wv,wa]);
    end
    
    R1 = diag(wu*ones(N,1));
    R2 = diag(wdu*ones(N-1,1));
    
    
    H = 2*(R1+S1'*Q*S1+D'*R2*D);
    f = 2*(T*x0+S2*V)'*Q*S1;
    
    u0 = zeros(N,1);
    options = optimoptions('quadprog','Algorithm','active-set');
    u_star = quadprog(H,f,A1,b1,Aeq,beq,lbu,ubu,u0,options);
DesiredAccel = u_star(1);

== stateflow chart BestRun_VehicleModel_pntwo/Following Vehicle (FV)/VehicleModel/shift_logic1 ==
  settings: sampleTime=0.005
  state gear_state [parallel]
    settings: executionOrder=1
    state five
      entry: gear = 5;
    state fourth
      entry: gear = 4;
    state third
      entry: gear = 3;
    state second
      entry: gear = 2;
    state first
      entry: gear = 1;
    fourth -> five [order 1] : UP
    (default) -> first
    second -> third [order 1] : UP
    first -> second : UP
    third -> fourth [order 1] : UP
    five -> fourth : DOWN
    third -> second [order 2] : DOWN
    fourth -> third [order 2] : DOWN
    second -> first [order 2] : DOWN
  state selection_state [parallel]
    during: CALC_TH;
    settings: executionOrder=2
    state steady_state
    state upshifting
    state downshifting
    (default) -> steady_state
    steady_state -> upshifting [order 1] : [speed > up_th]
    steady_state -> downshifting [order 2] : [speed < down_th]
    downshifting -> steady_state [order 1] : after(TWAIT,tick)
        | [speed <= down_th]
        | {gear_state.DOWN;}
    downshifting -> steady_state [order 2] : [speed > down_th]
    upshifting -> steady_state [order 1] : after(TWAIT,tick)
        | [speed >= up_th]
        | {gear_state.UP;}
    upshifting -> steady_state [order 2] : [speed < up_th]
  data: throttle input double; speed input double; gear output uint8 [1..5]; TWAIT parameter uint8; up_th input double; down_th input double
  events: DOWN local EITHER_EDGE_EVENT; UP local EITHER_EDGE_EVENT; CALC_TH output FUNCTION_CALL_EVENT
